simulink model "Lab3Transmitter"  (R2021b)
settings: Solver=VariableStepAuto  StartTime=0.0  StopTime=inf  RelTol=1e-3
undefined symbols (not defined in the file): frsTxCTCSSToneFrequencies, frsTxParams, frsTxSourceFrameLength, frsTxSourceSampleRate, Fs, ip, usb
libraries: dspmlti4 x2, dspsrcs4 x2, plutoradiolib x1, commanabbnd3 x1, dspvision x1
settings Model: Creator=keven  LastModifiedBy=Dlope

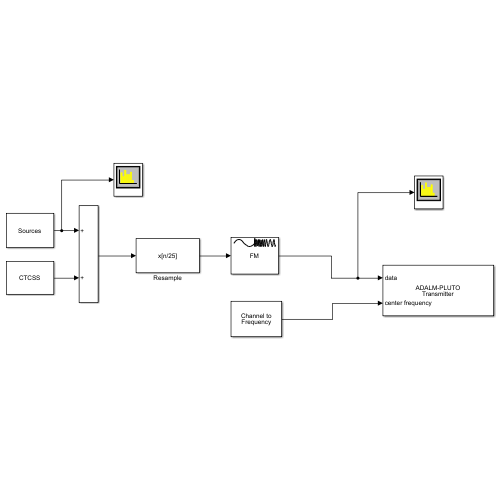
[thumbnail: Simulink's stored preview of the top-level diagram]
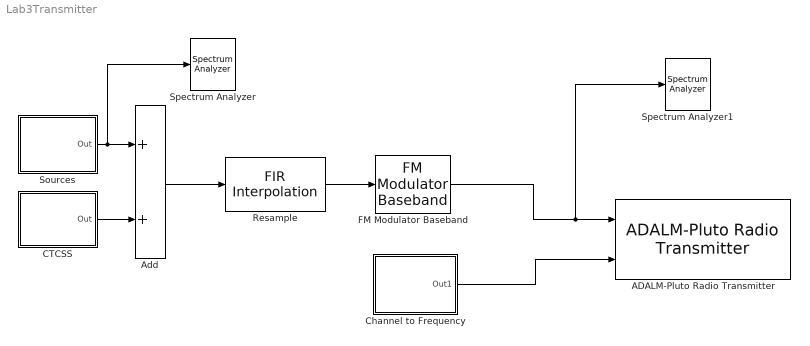
== system Lab3Transmitter ==
  ADALM-Pluto Radio Transmitter : plutoradiolib/ADALM-Pluto Radio Transmitter  RadioID=usb:0  uri=ip:10.0.0.200  CenterFrequencySource=Input Port  CenterFrequency=2.4e9  GainSource=Dialog  Gain=-15  ChannelMapping=1  BasebandSampleRate=200000  UnderflowOutputPort=off  ShowAdvancedProperties=off  UseCustomFilter=off  filtPathRates=[737280000 11520000 3840000 1920000 960000 240000]  filtCoefficients=[-192 82 85 -215 228 -102 -110 290 -318 145 160 -426 471 -215 -238 633 -697 318 349 -923 1009 -457 -498 1309 -1423 640 693 -1812 1959 -876 -945 2458 -2647 1180 1268 -3290 3534 -1572 -1688 4375 -4698 2091 2247 -5836 6284 -2807 -3031 7918 -8588 3870 4225 -11182 12324 -5662 -6330 17255 -19735 9507 11312 -33568 43355 -25227 -42139 305542 305542 -42139 -25227 43355 -33568 11312 9507 -19735 17255 -6330 -5662 12324 -11182 4225 3870 -8588 7918 -3031 -2807 6284 -5836 2247 2091 -4698 4375 -1688 -1572 3534 -3290 1268 1180 -2647 2458 -945 -876 1959 -1812 693 640 -1423 1309 -498 -457 1009 -923 349 318 -697 633 -238 -215 471 -426 160 145 -318 290 -110 -102 228 -215 85 82 -192]  filtCoefficientSize=128  filtDecimInterpFactor=4  filtGain=-12  filtRFBandwidth=18000000  filterConfigStruct=struct()  DataSourceSelect=Input Port  DDSTone1Freq=5e3  DDSTone2Freq=10e3  DDSTone1Scale=0.5  DDSTone2Scale=0.25  DataTimeout=Inf  FrequencyCorrection=0  ENSMPinControlMode=None  BISTLoopbackMode=Disabled  BISTToneInject=Disabled  BISTSignalGen=PRBS  BISTToneFreq=Fs/32  BISTToneLevel=0
      settings: SourceProductBaseCode=PLUTO
  Add : Sum
  CTCSS : Subsystem
      mask Display: disp('CTCSS')
  Channel to Frequency : Subsystem
      mask Display: disp('Channel to\nFrequency');
  FM Modulator Baseband : commanabbnd3/FM Modulator Baseband  FrequencyDeviation=2500  SimulateUsing=Code generation
      settings: SourceProductBaseCode=CM
  Resample : dspmlti4/FIR Interpolation  FilterSource=Auto  PrivateCoeffs=0  h=frsTxParams.InterpolationNumerator  L=25  FilterObject=FINTERP  InputProcessing=Columns as channels (frame based)  framing=Enforce single-rate processing  outputBufInitCond=0  roundingMode=Floor  overflowMode=off  firstCoeffDataTypeStr=Inherit: Same word length as input  firstCoeffMin=[]  firstCoeffMax=[]  firstCoeffLastDataTypeStr=Inherit: Same word length as input  outputDataTypeStr=Inherit: Same as accumulator  outputMin=[]  outputMax=[]  outputLastDataTypeStr=Inherit: Same as accumulator
  Sources : Subsystem
      mask Display: disp('Sources');
  Spectrum Analyzer : SpectrumAnalyzer
  Spectrum Analyzer1 : SpectrumAnalyzer
  wires:
  Add/1 -> Resample/1
  Sources/1(Out) -> Spectrum Analyzer/1, Add/1
  CTCSS/1(Out) -> Add/2
  FM Modulator Baseband/1 -> Spectrum Analyzer1/1, ADALM-Pluto Radio Transmitter/1
  Resample/1 -> FM Modulator Baseband/1
  Channel to Frequency/1(Out1) -> ADALM-Pluto Radio Transmitter/2

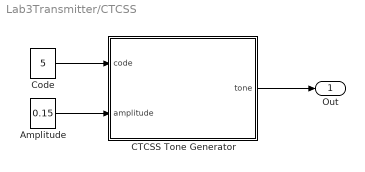
== system Lab3Transmitter/CTCSS ==
  Amplitude : Constant  Value=0.15  VectorParams1D=off  OutDataTypeStr=single  FramePeriod=-1
  CTCSS Tone Generator : MATLAB Function  TreatAsAtomicUnit=on
  Code : Constant  Value=5  VectorParams1D=off  OutDataTypeStr=uint8  FramePeriod=-1
  Out : Outport  VectorParamsAs1DForOutWhenUnconnected=off
  wires:
  Code/1 -> CTCSS Tone Generator/1(code)
  Amplitude/1 -> CTCSS Tone Generator/2(amplitude)
  CTCSS Tone Generator/1(tone) -> Out/1

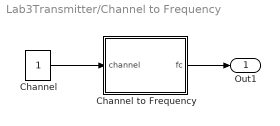
== system Lab3Transmitter/Channel to Frequency ==
  Channel : Constant  VectorParams1D=off  OutDataTypeStr=uint8  FramePeriod=-1
  Channel to Frequency : MATLAB Function  TreatAsAtomicUnit=on
  Out1 : Outport  VectorParamsAs1DForOutWhenUnconnected=off
  wires:
  Channel/1 -> Channel to Frequency/1(channel)
  Channel to Frequency/1(fc) -> Out1/1

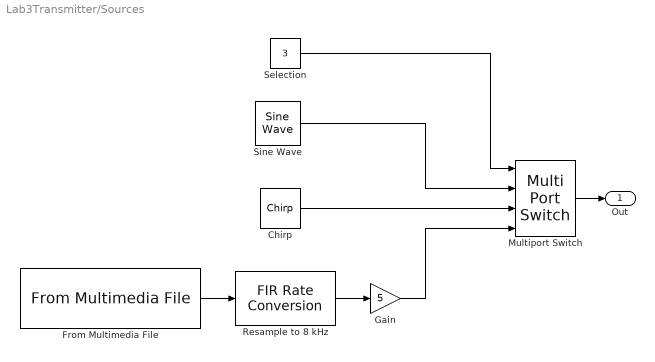
== system Lab3Transmitter/Sources ==
  " Resample to 8 kHz" : dspmlti4/FIR Rate Conversion  FilterSource=Auto  L=160  h=[1 1]  M=441  FilterObject=FRC  rateMode=Enforce single-rate processing  roundingMode=Floor  overflowMode=off  firstCoeffDataTypeStr=Inherit: Same word length as input  firstCoeffMin=[]  firstCoeffMax=[]  firstCoeffLastDataTypeStr=Inherit: Same word length as input  outputDataTypeStr=Inherit: Same as accumulator  outputMin=[]  outputMax=[]  outputLastDataTypeStr=Inherit: Same as accumulator
      settings: SourceProductBaseCode=DS
  Chirp : dspsrcs4/Chirp  sweep=Linear  mode=Unidirectional  f0=600  f1=1200  t1=3  Tsweep=3  phase=0  Ts=1/frsTxParams.SourceSampleRate  spf=frsTxParams.SourceFrameLength  datatype=Single  OutputFrames=off
  From Multimedia File : dspvision/From Multimedia File  inputFilename=C:\Users\Dlope\OneDrive - University of Massachusetts Dartmouth\Desktop\CantinaBand60.wav  readRange=[1 Inf]  loop=on  numPlays=inf  outputStreams=Audio only  videoDataType=single  audioDataType=single  inheritSampleTime=on  userDefinedSampleTime=1/30  noAudioOutput=off  isIntensityVideo=off  fourcc=RGB  colorVideoFormat=Separate color signals  outputEOF=off  dataOrg=Column-major  audioFrameSize=frsTxParams.AudioFrameLength  computeAudioFrameSize=off  outSamplingMode=Sample based
  Gain : Gain  Gain=5
  Multiport Switch : MultiPortSwitch
  Selection : Constant  Value=3
  Sine Wave : dspsrcs4/Sine Wave  Amplitude=1  Frequency=880  Phase=0  SampleMode=Discrete  OutComplex=Real  CompMethod=Trigonometric fcn  TableSize=Speed  SampleTime=1/frsTxParams.SourceSampleRate  SamplesPerFrame=frsTxParams.SourceFrameLength  ResetState=Restart at time zero  OutputFrames=off  dataType=single  wordLen=16  udDataType=sfix(16)  fracBitsMode=Best precision  numFracBits=15  OutDataTypeStr=single  LastOutDataTypeStr=single
  Out : Outport  VectorParamsAs1DForOutWhenUnconnected=off
  wires:
  From Multimedia File/1 -> " Resample to 8 kHz"/1
  Sine Wave/1 -> Multiport Switch/2
  " Resample to 8 kHz"/1 -> Gain/1
  Chirp/1 -> Multiport Switch/3
  Selection/1 -> Multiport Switch/1
  Multiport Switch/1 -> Out/1
  Gain/1 -> Multiport Switch/4

== matlab function Lab3Transmitter/CTCSS/CTCSS Tone Generator ==
  data: code input; tone output size=[frsTxSourceFrameLength, 1]; amplitude input; frsTxCTCSSToneFrequencies parameter; frsTxSourceSampleRate parameter; frsTxSourceFrameLength parameter
function tone  = CTCSS_Gen(code, amplitude, frsTxCTCSSToneFrequencies, ...
    frsTxSourceSampleRate, frsTxSourceFrameLength)
%#codegen

% Generate continuous phase sine wave
%
% PL   Hz     PL   Hz      PL   Hz
% --  ----    --  -----    --  -----
%  1  67.0    12  100.0    32  203.5
%  2  71.9    13  103.5    33  210.7
%  3  74.4    14  107.2    34  218.1
%  4  77.0    15  110.9    35  225.7
%  5  79.7    16  114.8    36  233.6
%  6  82.5    17  118.8    37  241.8
%  7  85.4    18  123.0    38  250.3
%  8  88.5    19  127.3
%  9  91.5    20  131.8
% 10  94.8    21  136.5
% 11  97.4    22  141.3
%             23  146.2
%             24  151.4
%             25  156.7
%             26  162.2
%             27  167.9
%             28  173.8
%             29  179.9
%             30  186.2
%             31  192.8

persistent t0 % The starting time of each frame

Freq = frsTxCTCSSToneFrequencies(code);

if isempty(t0)
    t0 = 0;
end

t = t0 + (0: frsTxSourceFrameLength-1) / frsTxSourceSampleRate;

t0 = t0 + frsTxSourceFrameLength/frsTxSourceSampleRate; % The starting time for the next frame

% wrap the time within the first period of the sine wave
if (t0 > 1/Freq)
    t0 = mod(t0, 1/Freq);
end

tone = single(single(amplitude) * sin(2*pi*Freq*t))';

== matlab function Lab3Transmitter/Channel to Frequency/Channel to Frequency ==
  data: channel input uint8; fc output double
function fc = ChanToFreq(channel)
%#codegen
% Map integer channel number to FRS/GMRS center frequencies

fc = convertChan2FreqFRSGMRSDemo(channel);
